simulink model "model"  (R2024a)
settings: Solver=VariableStepAuto  StartTime=0.0  StopTime=10.0  RelTol=1e-3
settings Model: Creator=Abhishek Gonnade  LastModifiedBy=Abhishek Gonnade

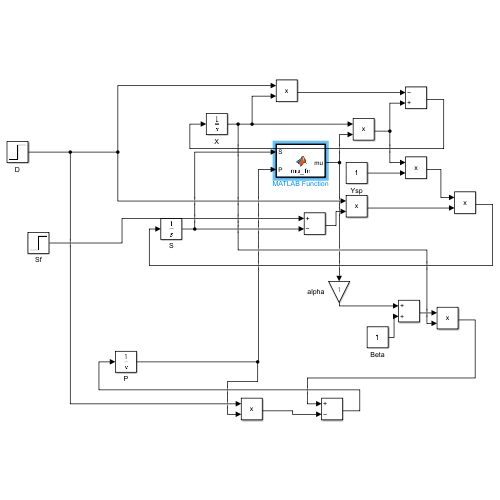
[thumbnail: Simulink's stored preview of the top-level diagram]
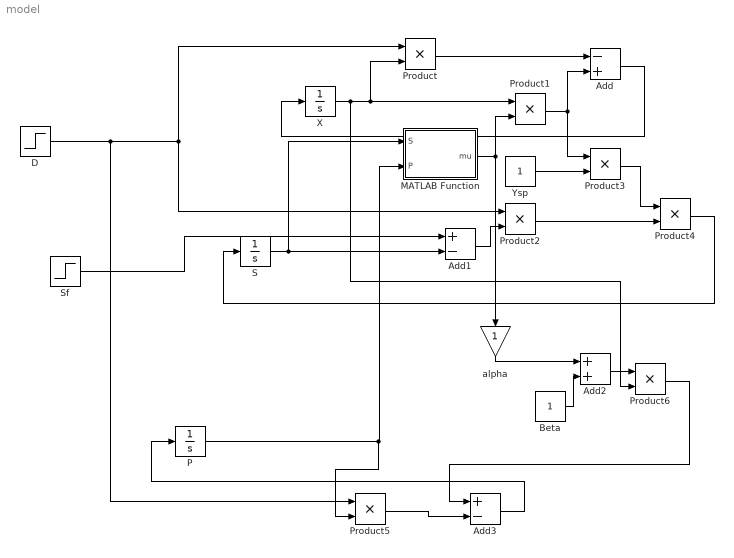
== system model ==
  Add : Sum  Inputs=-+
  Add1 : Sum  Inputs=+-
  Add2 : Sum
  Add3 : Sum  Inputs=+-
  Beta : Constant
  D : Step  Time=100  Before=0.202  After=0.202  SampleTime=1
  MATLAB Function : MATLAB Function  TreatAsAtomicUnit=on
  P : Integrator  InitialCondition=0.1
  Product{,1..6} (7 alike) : Product
  S : Integrator  InitialCondition=0.1
  Sf : Step  Time=100  Before=20  After=20  SampleTime=1
  X : Integrator  InitialCondition=0.1
  Ysp : Constant
  alpha : Gain
  wires:
  X/1 -> Product6/2, Product1/1, Product/2
  D/1 -> Product5/1, Product2/1, Product/1
  P/1 -> Product5/2, MATLAB Function/2(P)
  MATLAB Function/1(mu) -> alpha/1, Product1/2
  Product/1 -> Add/1
  Product1/1 -> Product3/1, Add/2
  Add/1 -> X/1
  Sf/1 -> Add1/1
  S/1 -> MATLAB Function/1(S), Add1/2
  Add1/1 -> Product2/2
  Ysp/1 -> Product3/2
  Product3/1 -> Product4/1
  Product2/1 -> Product4/2
  Product4/1 -> S/1
  alpha/1 -> Add2/1
  Beta/1 -> Add2/2
  Add2/1 -> Product6/1
  Product5/1 -> Add3/2
  Product6/1 -> Add3/1
  Add3/1 -> P/1

== matlab function model/MATLAB Function ==
  data: S input; mu output; P input
function mu = mu_fn(S, P)
    u_m = 0.48;
    P_m = 50;
    K_m = 1.2;
    S_f = 20;
    
end
